simulink model "CombinedVehicleModel"  (R2019a)
settings: Solver=VariableStepAuto  StartTime=0.0  StopTime=50  RelTol=1e-3
values from neighbouring files (symbols this model uses):
  a = 1.2    [Part33DofPar.m]    (also in Part3BicyclePar.m; part23.m)
  b = 1.4    [Part33DofPar.m]    (also in Part3BicyclePar.m; part23.m)
  caf = 25000    [Part33DofPar.m]    (also in Part3BicyclePar.m = 50000; part23.m)
  car = 25000    [Part33DofPar.m]    (also in Part3BicyclePar.m = 50000; part23.m)
  Iz = 2000    [Part33DofPar.m]    (also in Part3BicyclePar.m; part23.m)
  M = 1000    [Part33DofPar.m]    (also in Part3BicyclePar.m; part23.m)
  tr = 10/180*pi    (= 0.174532925199)    [Part3BicyclePar.m]
undefined symbols (not defined in the file or in its folder): T
libraries: simulink x1
settings Model: Creator=a33shahi  LastModifiedBy=a33shahi

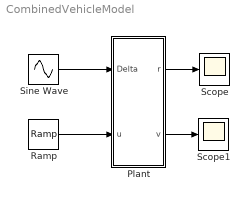
== system CombinedVehicleModel ==
  Plant : Subsystem
  Ramp : simulink/Sources/Ramp  slope=20/50  start=0  InitialOutput=1
  Scope : Scope
  Scope1 : Scope
  Sine Wave : Sin  Amplitude=6*pi/180  SampleTime=0
  wires:
  Sine Wave/1 -> Plant/1(Delta)
  Ramp/1 -> Plant/2(u)
  Plant/1(r) -> Scope/1
  Plant/2(v) -> Scope1/1

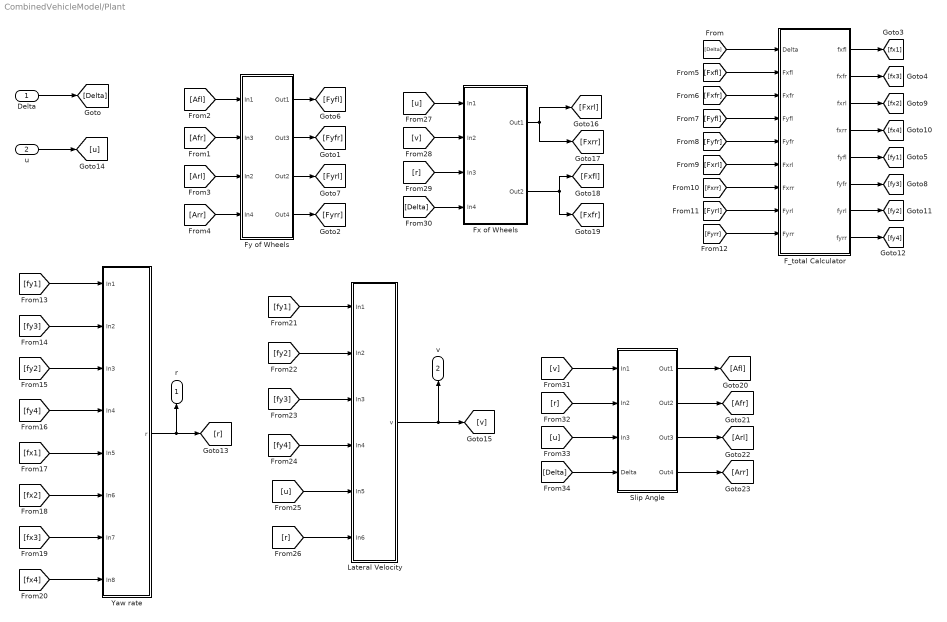
== system CombinedVehicleModel/Plant ==
  Delta : Inport
  u : Inport  Port=2
  F_total Calculator : Subsystem
  Fx of Wheels : Subsystem
  Fy of Wheels : Subsystem
  Lateral Velocity : Subsystem
  Slip Angle : Subsystem
  Yaw rate : Subsystem
  r : Outport
  v : Outport  Port=2
  wires:
  [Arr] -> Fy of Wheels/4(In4)
  [u] -> Fx of Wheels/1(In1)
  F_total Calculator/7(fyrl) -> [fy2]
  Slip Angle/3(Out3) -> [Arl]
  [Fyrl] -> F_total Calculator/8(Fyrl)
  [Fyfl] -> F_total Calculator/4(Fyfl)
  [v] -> Fx of Wheels/2(In2)
  [Fyfr] -> F_total Calculator/5(Fyfr)
  F_total Calculator/6(fyfr) -> [fy3]
  [Delta] -> Fx of Wheels/4(In4)
  [Fxfr] -> F_total Calculator/3(Fxfr)
  [r] -> Fx of Wheels/3(In3)
  Fx of Wheels/1(Out1) -> [Fxrl], [Fxrr]
  F_total Calculator/2(fxfr) -> [fx3]
  Fx of Wheels/2(Out2) -> [Fxfl], [Fxfr]
  [Afr] -> Fy of Wheels/2(In3)
  [Fyrr] -> F_total Calculator/9(Fyrr)
  [fx1] -> Yaw rate/5(In5)
  [Fxrl] -> F_total Calculator/6(Fxrl)
  Yaw rate/1(r) -> r/1, [r]
  Delta/1 -> [Delta]
  F_total Calculator/8(fyrr) -> [fy4]
  [Delta] -> F_total Calculator/1(Delta)
  Fy of Wheels/4(Out4) -> [Fyrr]
  F_total Calculator/5(fyfl) -> [fy1]
  F_total Calculator/1(fxfl) -> [fx1]
  Fy of Wheels/2(Out3) -> [Fyfr]
  Fy of Wheels/3(Out2) -> [Fyrl]
  [fx3] -> Yaw rate/7(In7)
  [fy4] -> Yaw rate/4(In4)
  [fy2] -> Lateral Velocity/2(In2)
  Fy of Wheels/1(Out1) -> [Fyfl]
  Lateral Velocity/1(v) -> [v], v/1
  [Arl] -> Fy of Wheels/3(In2)
  [fy4] -> Lateral Velocity/4(In4)
  [Afl] -> Fy of Wheels/1(In1)
  F_total Calculator/3(fxrl) -> [fx2]
  u/1 -> [u]
  [fx2] -> Yaw rate/6(In6)
  [Fxfl] -> F_total Calculator/2(Fxfl)
  [fy2] -> Yaw rate/3(In3)
  [Fxrr] -> F_total Calculator/7(Fxrr)
  [fy1] -> Yaw rate/1(In1)
  F_total Calculator/4(fxrr) -> [fx4]
  [fy3] -> Yaw rate/2(In2)
  [fx4] -> Yaw rate/8(In8)
  [fy3] -> Lateral Velocity/3(In3)
  Slip Angle/4(Out4) -> [Arr]
  [fy1] -> Lateral Velocity/1(In1)
  [u] -> Lateral Velocity/5(In5)
  [r] -> Lateral Velocity/6(In6)
  [v] -> Slip Angle/1(In1)
  [u] -> Slip Angle/3(In3)
  Slip Angle/1(Out1) -> [Afl]
  [r] -> Slip Angle/2(In2)
  Slip Angle/2(Out2) -> [Afr]
  [Delta] -> Slip Angle/4(Delta)

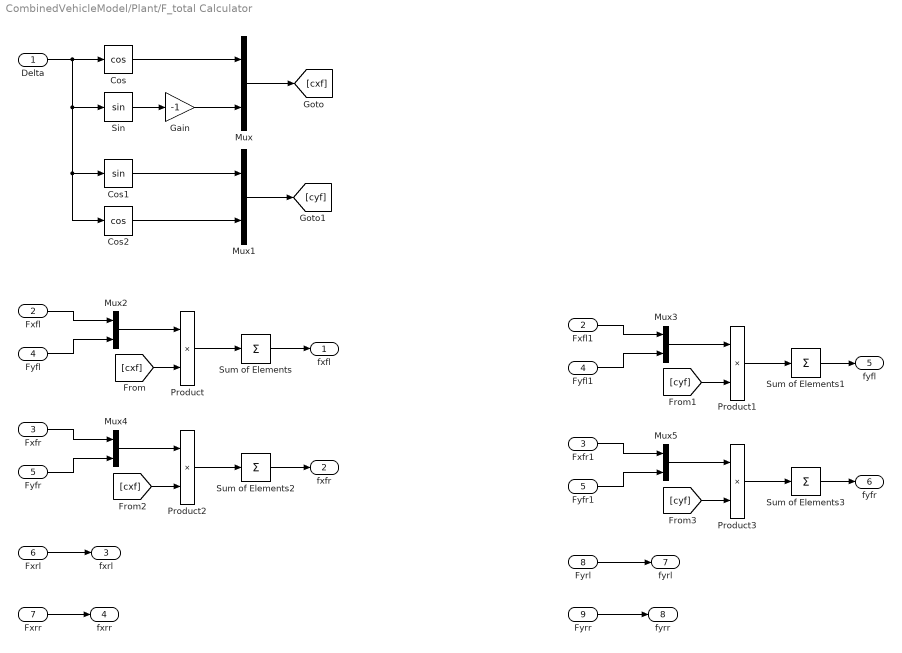
== system CombinedVehicleModel/Plant/F_total Calculator ==
  Delta : Inport
  Fxfl : Inport  Port=2
  Fxfr : Inport  Port=3
  Fyfl : Inport  Port=4
  Fyfr : Inport  Port=5
  Fxrl : Inport  Port=6
  Fxrr : Inport  Port=7
  Fyrl : Inport  Port=8
  Fyrr : Inport  Port=9
  Cos : Trigonometry  Operator=cos
  Cos1 : Trigonometry
  Cos2 : Trigonometry  Operator=cos
  Fxfl1 : InportShadow  Port=2
  Fxfr1 : InportShadow  Port=3
  Fyfl1 : InportShadow  Port=4
  Fyfr1 : InportShadow  Port=5
  Gain : Gain  Gain=-1
  Mux{,1..5} (6 alike) : Mux  Inputs=2
  Product{,1..3} (4 alike) : Product
  Sin : Trigonometry
  Sum of Elements{,1..3} (4 alike) : Sum  Inputs=+
  fxfl : Outport
  fxfr : Outport  Port=2
  fxrl : Outport  Port=3
  fxrr : Outport  Port=4
  fyfl : Outport  Port=5
  fyfr : Outport  Port=6
  fyrl : Outport  Port=7
  fyrr : Outport  Port=8
  wires:
  Cos/1 -> Mux/1
  Sin/1 -> Gain/1
  Gain/1 -> Mux/2
  Mux/1 -> [cxf]
  Mux1/1 -> [cyf]
  Cos2/1 -> Mux1/2
  Cos1/1 -> Mux1/1
  Delta/1 -> Cos2/1, Cos1/1, Sin/1, Cos/1
  Fxfl/1 -> Mux2/1
  Fyfl/1 -> Mux2/2
  Mux2/1 -> Product/1
  [cxf] -> Product/2
  Product/1 -> Sum of Elements/1
  Sum of Elements/1 -> fxfl/1
  Sum of Elements2/1 -> fxfr/1
  Product2/1 -> Sum of Elements2/1
  [cxf] -> Product2/2
  Mux4/1 -> Product2/1
  Fyfr/1 -> Mux4/2
  Fxfr/1 -> Mux4/1
  Fxrl/1 -> fxrl/1
  Fxrr/1 -> fxrr/1
  Fxfr1/1 -> Mux5/1
  Fyfr1/1 -> Mux5/2
  Mux5/1 -> Product3/1
  [cyf] -> Product3/2
  Product3/1 -> Sum of Elements3/1
  Sum of Elements3/1 -> fyfr/1
  Sum of Elements1/1 -> fyfl/1
  Product1/1 -> Sum of Elements1/1
  [cyf] -> Product1/2
  Mux3/1 -> Product1/1
  Fyfl1/1 -> Mux3/2
  Fxfl1/1 -> Mux3/1
  Fyrl/1 -> fyrl/1
  Fyrr/1 -> fyrr/1

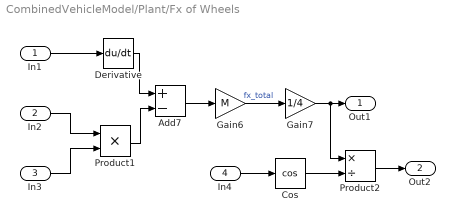
== system CombinedVehicleModel/Plant/Fx of Wheels ==
  In1 : Inport
  In2 : Inport  Port=2
  In3 : Inport  Port=3
  In4 : Inport  Port=4
  Add7 : Sum  Inputs=+-
  Cos : Trigonometry  Operator=cos
  Derivative : Derivative
  Gain6 : Gain  Gain=M
  Gain7 : Gain  Gain=1/4
  Product1 : Product
  Product2 : Product  Inputs=*/
  Out1 : Outport
  Out2 : Outport  Port=2
  wires:
  Gain6/1 -> Gain7/1  "fx_total"
  Gain7/1 -> Product2/1, Out1/1
  Add7/1 -> Gain6/1
  Cos/1 -> Product2/2
  Product1/1 -> Add7/2
  In4/1 -> Cos/1
  Derivative/1 -> Add7/1
  In1/1 -> Derivative/1
  In2/1 -> Product1/1
  Product2/1 -> Out2/1
  In3/1 -> Product1/2

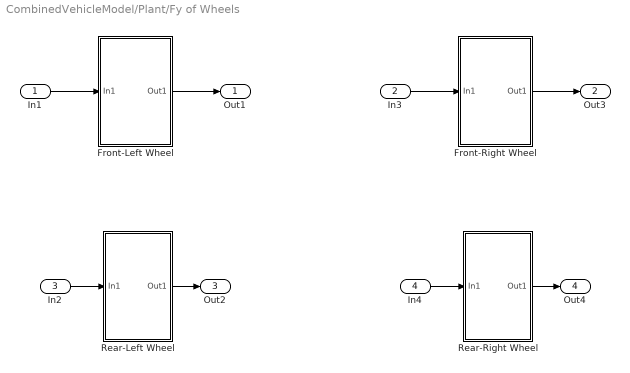
== system CombinedVehicleModel/Plant/Fy of Wheels ==
  In1 : Inport
  In3 : Inport  Port=2
  In2 : Inport  Port=3
  In4 : Inport  Port=4
  Front-Left Wheel : Subsystem
  Front-Right Wheel : Subsystem
  Rear-Left Wheel : Subsystem
  Rear-Right Wheel : Subsystem
  Out1 : Outport
  Out3 : Outport  Port=2
  Out2 : Outport  Port=3
  Out4 : Outport  Port=4
  wires:
  In1/1 -> Front-Left Wheel/1(In1)
  Front-Left Wheel/1(Out1) -> Out1/1
  In2/1 -> Rear-Left Wheel/1(In1)
  Rear-Left Wheel/1(Out1) -> Out2/1
  Rear-Right Wheel/1(Out1) -> Out4/1
  In4/1 -> Rear-Right Wheel/1(In1)
  Front-Right Wheel/1(Out1) -> Out3/1
  In3/1 -> Front-Right Wheel/1(In1)

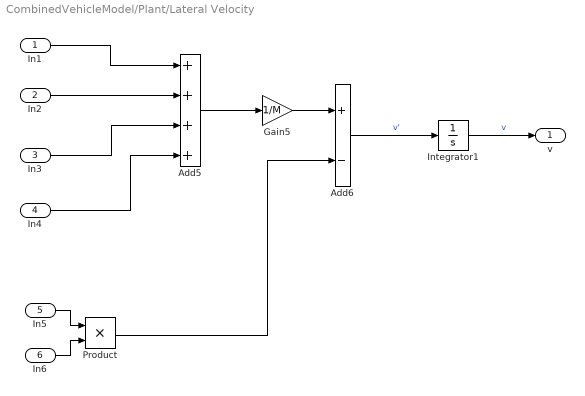
== system CombinedVehicleModel/Plant/Lateral Velocity ==
  In1 : Inport
  In2 : Inport  Port=2
  In3 : Inport  Port=3
  In4 : Inport  Port=4
  In5 : Inport  Port=5
  In6 : Inport  Port=6
  Add5 : Sum  Inputs=++++
  Add6 : Sum  Inputs=+-
  Gain5 : Gain  Gain=1/M
  Integrator1 : Integrator
  Product : Product
  v : Outport
  wires:
  Gain5/1 -> Add6/1
  In5/1 -> Product/1
  Product/1 -> Add6/2
  In3/1 -> Add5/3
  In4/1 -> Add5/4
  In1/1 -> Add5/1
  Add5/1 -> Gain5/1
  Add6/1 -> Integrator1/1  "v'"
  In6/1 -> Product/2
  In2/1 -> Add5/2
  Integrator1/1 -> v/1  "v"

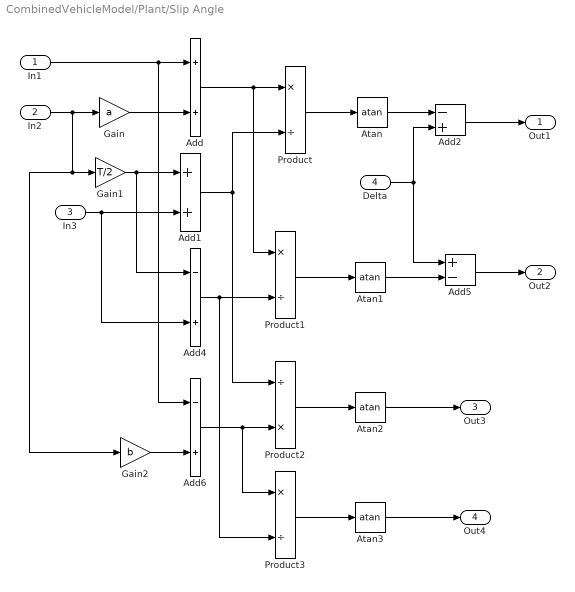
== system CombinedVehicleModel/Plant/Slip Angle ==
  In1 : Inport
  In2 : Inport  Port=2
  In3 : Inport  Port=3
  Delta : Inport  Port=4
  Add : Sum
  Add1 : Sum
  Add2 : Sum  Inputs=-+
  Add4 : Sum  Inputs=-+
  Add5 : Sum  Inputs=+-
  Add6 : Sum  Inputs=-+
  Atan{,1..3} (4 alike) : Trigonometry  Operator=atan
  Gain : Gain  Gain=a
  Gain1 : Gain  Gain=T/2
  Gain2 : Gain  Gain=b
  Product : Product  Inputs=*/
  Product1 : Product  Inputs=*/
  Product2 : Product  Inputs=/*
  Product3 : Product  Inputs=*/
  Out1 : Outport
  Out2 : Outport  Port=2
  Out3 : Outport  Port=3
  Out4 : Outport  Port=4
  wires:
  Atan/1 -> Add2/1
  Add/1 -> Product1/1, Product/1
  Product2/1 -> Atan2/1
  Atan2/1 -> Out3/1
  In2/1 -> Gain2/1, Gain1/1, Gain/1
  Gain/1 -> Add/2
  Add1/1 -> Product/2, Product2/1
  Product/1 -> Atan/1
  Add4/1 -> Product3/2, Product1/2
  Add2/1 -> Out1/1
  Product1/1 -> Atan1/1
  In1/1 -> Add6/1, Add/1
  Gain2/1 -> Add6/2
  Add6/1 -> Product3/1, Product2/2
  In3/1 -> Add4/2, Add1/2
  Product3/1 -> Atan3/1
  Gain1/1 -> Add4/1, Add1/1
  Atan1/1 -> Add5/2
  Delta/1 -> Add2/2, Add5/1
  Atan3/1 -> Out4/1
  Add5/1 -> Out2/1

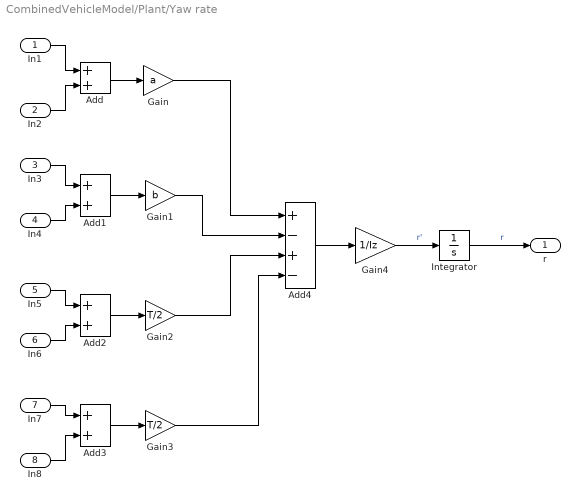
== system CombinedVehicleModel/Plant/Yaw rate ==
  In1 : Inport
  In2 : Inport  Port=2
  In3 : Inport  Port=3
  In4 : Inport  Port=4
  In5 : Inport  Port=5
  In6 : Inport  Port=6
  In7 : Inport  Port=7
  In8 : Inport  Port=8
  Add{,1..3} (4 alike) : Sum
  Add4 : Sum  Inputs=+-+-
  Gain : Gain  Gain=a
  Gain1 : Gain  Gain=b
  Gain2 : Gain  Gain=T/2
  Gain3 : Gain  Gain=T/2
  Gain4 : Gain  Gain=1/Iz
  Integrator : Integrator
  r : Outport
  wires:
  Add3/1 -> Gain3/1
  In3/1 -> Add1/1
  Add/1 -> Gain/1
  Add1/1 -> Gain1/1
  Gain2/1 -> Add4/3
  Gain1/1 -> Add4/2
  In2/1 -> Add/2
  Gain3/1 -> Add4/4
  Add4/1 -> Gain4/1
  In4/1 -> Add1/2
  Gain/1 -> Add4/1
  Add2/1 -> Gain2/1
  Gain4/1 -> Integrator/1  "r'"
  Integrator/1 -> r/1  "r"
  In1/1 -> Add/1
  In6/1 -> Add2/2
  In5/1 -> Add2/1
  In8/1 -> Add3/2
  In7/1 -> Add3/1

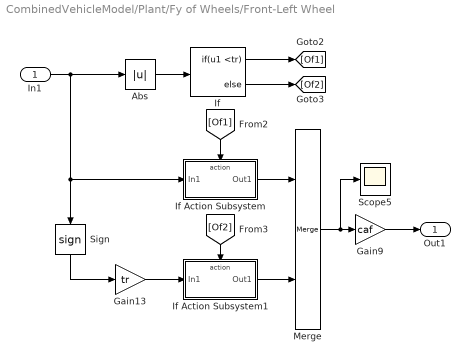
== system CombinedVehicleModel/Plant/Fy of Wheels/Front-Left Wheel ==
  In1 : Inport
  Abs : Abs
  Gain13 : Gain  Gain=tr
  Gain9 : Gain  Gain=caf
  If : If  IfExpression=u1 <tr
  If Action Subsystem : Subsystem  TreatAsAtomicUnit=on
  If Action Subsystem1 : Subsystem  TreatAsAtomicUnit=on
  Merge : Merge
  Scope5 : Scope
  Sign : Signum
  Out1 : Outport
  wires:
  If Action Subsystem1/1(Out1) -> Merge/2
  Abs/1 -> If/1
  [Of1] -> If Action Subsystem/Action
  If/1 -> [Of1]
  If/2 -> [Of2]
  Merge/1 -> Scope5/1, Gain9/1
  In1/1 -> If Action Subsystem/1(In1), Sign/1, Abs/1
  If Action Subsystem/1(Out1) -> Merge/1
  Sign/1 -> Gain13/1
  [Of2] -> If Action Subsystem1/Action
  Gain13/1 -> If Action Subsystem1/1(In1)
  Gain9/1 -> Out1/1

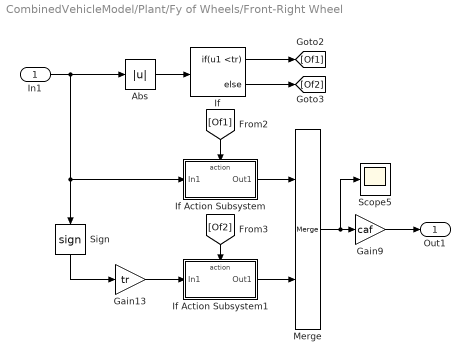
== system CombinedVehicleModel/Plant/Fy of Wheels/Front-Right Wheel ==
  In1 : Inport
  Abs : Abs
  Gain13 : Gain  Gain=tr
  Gain9 : Gain  Gain=caf
  If : If  IfExpression=u1 <tr
  If Action Subsystem : Subsystem  TreatAsAtomicUnit=on
  If Action Subsystem1 : Subsystem  TreatAsAtomicUnit=on
  Merge : Merge
  Scope5 : Scope
  Sign : Signum
  Out1 : Outport
  wires:
  Gain9/1 -> Out1/1
  Gain13/1 -> If Action Subsystem1/1(In1)
  [Of2] -> If Action Subsystem1/Action
  Sign/1 -> Gain13/1
  If Action Subsystem/1(Out1) -> Merge/1
  In1/1 -> Abs/1, Sign/1, If Action Subsystem/1(In1)
  Merge/1 -> Gain9/1, Scope5/1
  If/2 -> [Of2]
  If/1 -> [Of1]
  [Of1] -> If Action Subsystem/Action
  Abs/1 -> If/1
  If Action Subsystem1/1(Out1) -> Merge/2

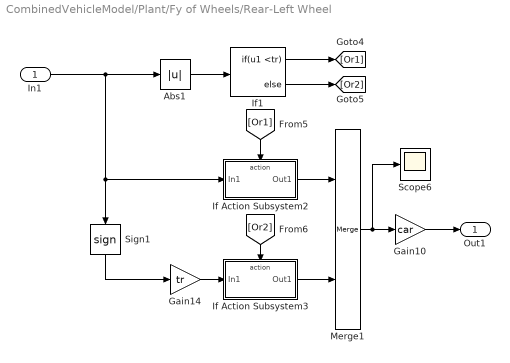
== system CombinedVehicleModel/Plant/Fy of Wheels/Rear-Left Wheel ==
  In1 : Inport
  Abs1 : Abs
  Gain10 : Gain  Gain=car
  Gain14 : Gain  Gain=tr
  If Action Subsystem2 : Subsystem  TreatAsAtomicUnit=on
  If Action Subsystem3 : Subsystem  TreatAsAtomicUnit=on
  If1 : If  IfExpression=u1 <tr
  Merge1 : Merge
  Scope6 : Scope
  Sign1 : Signum
  Out1 : Outport
  wires:
  [Or2] -> If Action Subsystem3/Action
  Gain14/1 -> If Action Subsystem3/1(In1)
  If1/2 -> [Or2]
  Sign1/1 -> Gain14/1
  Merge1/1 -> Scope6/1, Gain10/1
  If1/1 -> [Or1]
  In1/1 -> Sign1/1, If Action Subsystem2/1(In1), Abs1/1
  If Action Subsystem2/1(Out1) -> Merge1/1
  [Or1] -> If Action Subsystem2/Action
  If Action Subsystem3/1(Out1) -> Merge1/2
  Abs1/1 -> If1/1
  Gain10/1 -> Out1/1

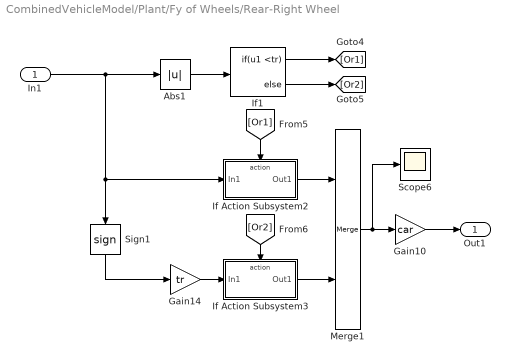
== system CombinedVehicleModel/Plant/Fy of Wheels/Rear-Right Wheel ==
  In1 : Inport
  Abs1 : Abs
  Gain10 : Gain  Gain=car
  Gain14 : Gain  Gain=tr
  If Action Subsystem2 : Subsystem  TreatAsAtomicUnit=on
  If Action Subsystem3 : Subsystem  TreatAsAtomicUnit=on
  If1 : If  IfExpression=u1 <tr
  Merge1 : Merge
  Scope6 : Scope
  Sign1 : Signum
  Out1 : Outport
  wires:
  Gain10/1 -> Out1/1
  Abs1/1 -> If1/1
  If Action Subsystem3/1(Out1) -> Merge1/2
  [Or1] -> If Action Subsystem2/Action
  If Action Subsystem2/1(Out1) -> Merge1/1
  In1/1 -> Abs1/1, If Action Subsystem2/1(In1), Sign1/1
  If1/1 -> [Or1]
  Merge1/1 -> Gain10/1, Scope6/1
  Sign1/1 -> Gain14/1
  If1/2 -> [Or2]
  Gain14/1 -> If Action Subsystem3/1(In1)
  [Or2] -> If Action Subsystem3/Action

== system CombinedVehicleModel/Plant/Fy of Wheels/Front-Left Wheel/If Action Subsystem ==
  In1 : Inport
  Action Port : ActionPort  ActionPortLabel=if(u1 <tr)
  Out1 : Outport
  wires:
  In1/1 -> Out1/1

== system CombinedVehicleModel/Plant/Fy of Wheels/Front-Left Wheel/If Action Subsystem1 ==
  In1 : Inport
  Action Port : ActionPort  ActionPortLabel=else
  Out1 : Outport
  wires:
  In1/1 -> Out1/1

== system CombinedVehicleModel/Plant/Fy of Wheels/Front-Right Wheel/If Action Subsystem ==
  In1 : Inport
  Action Port : ActionPort  ActionPortLabel=if(u1 <tr)
  Out1 : Outport
  wires:
  In1/1 -> Out1/1

== system CombinedVehicleModel/Plant/Fy of Wheels/Front-Right Wheel/If Action Subsystem1 ==
  In1 : Inport
  Action Port : ActionPort  ActionPortLabel=else
  Out1 : Outport
  wires:
  In1/1 -> Out1/1

== system CombinedVehicleModel/Plant/Fy of Wheels/Rear-Left Wheel/If Action Subsystem2 ==
  In1 : Inport
  Action Port : ActionPort  ActionPortLabel=if(u1 <tr)
  Out1 : Outport
  wires:
  In1/1 -> Out1/1

== system CombinedVehicleModel/Plant/Fy of Wheels/Rear-Left Wheel/If Action Subsystem3 ==
  In1 : Inport
  Action Port : ActionPort  ActionPortLabel=else
  Out1 : Outport
  wires:
  In1/1 -> Out1/1

== system CombinedVehicleModel/Plant/Fy of Wheels/Rear-Right Wheel/If Action Subsystem2 ==
  In1 : Inport
  Action Port : ActionPort  ActionPortLabel=if(u1 <tr)
  Out1 : Outport
  wires:
  In1/1 -> Out1/1

== system CombinedVehicleModel/Plant/Fy of Wheels/Rear-Right Wheel/If Action Subsystem3 ==
  In1 : Inport
  Action Port : ActionPort  ActionPortLabel=else
  Out1 : Outport
  wires:
  In1/1 -> Out1/1
